simulink model "TestReadData"  (R2023b)
settings: Solver=VariableStepAuto  StartTime=0.0  StopTime=10.0  RelTol=1e-3
settings Model: Creator=han  LastModifiedBy=han
settings DataIOCC: ExternalInput=p2

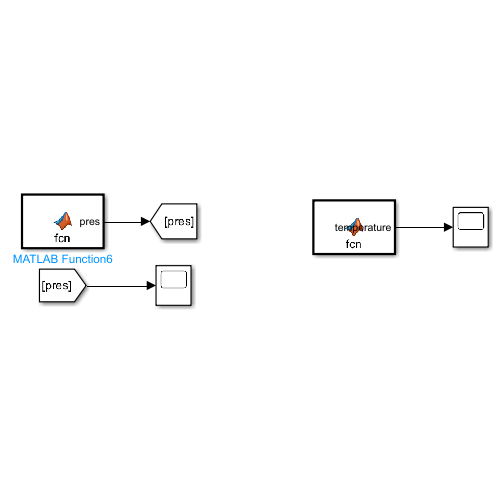
[thumbnail: Simulink's stored preview of the top-level diagram]
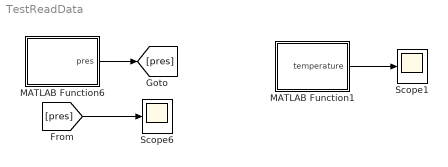
== system TestReadData ==
  MATLAB Function1 : MATLAB Function  TreatAsAtomicUnit=on
  MATLAB Function6 : MATLAB Function  TreatAsAtomicUnit=on
  Scope1 : Scope
  Scope6 : Scope
  wires:
  MATLAB Function6/1(pres) -> [pres]
  [pres] -> Scope6/1
  MATLAB Function1/1(temperature) -> Scope1/1

== matlab function TestReadData/MATLAB Function6 ==
  data: pres output
function pres = fcn()
coder.extrinsic("py.pyvista")
coder.extrinsic("py.numpy")
coder.extrinsic("py.ReadData.py")
coder.extrinsic("py.ReadData.get_pressure")
pres = 0.0;
pres = py.ReadData.get_pressure(8.14937,0.0,-0.92);

== matlab function TestReadData/MATLAB Function1 ==
  data: temperature output
function temperature = fcn()
coder.extrinsic("py.pyvista")
coder.extrinsic("py.numpy")
coder.extrinsic("py.ReadData.py")
coder.extrinsic("py.ReadData.get_temperature")
temperature = 0.0;
temperature = py.ReadData.get_temperature(8.14937,0.0,-0.92);
